simulink model "HIL_model_overall"  (R2014a)
settings: Solver=ode5  StartTime=0.0  StopTime=simulationTime  FixedStep=0.1  RelTol=1e-3
values from neighbouring files (symbols this model uses):
  A_ref = [0.176     0           0 ... (first row only)    [theProgram.m]
  B_ref = [0.0554     0           0 ... (first row only)    [theProgram.m]
  C_ref = [0.05*0.0038     0           0 ... (first row only)    [theProgram.m]
  Di = [50 0 ... (first row only)    [theProgram.m]
  Dist_spv_rfp = sqrt( ( shipL_d(1) - Rfp(1) )^2 + (shipL_d(2) - Rfp(2) )^2 )    [theProgram.m]
  Ds = [-X_u 0 0 ... (first row only)    [theProgram.m]
  iceDiameter = 0.2    [theProgram.m]
  K2_obs = diag([0.25 1 0.5])    [theProgram.m]
  K3_obs = diag([1 1 1])    [theProgram.m]
  K4_obs = diag([250 300 100])    [theProgram.m]
  K_M = [ 1 0 0 ... (first row only)    [theProgram.m]
  K_tow = 20    [theProgram.m]
  kappa = 2    [theProgram.m]
  Kd = [50 0 0 ... (first row only)    [theProgram.m]
  Kp = [10 0 0 ... (first row only)    [theProgram.m]
  Mi_a = iceMass*[1 0; 0 1]    [theProgram.m]
  Mi_rb = iceMass*[1 0; 0 1]    [theProgram.m]
  Ms_a = -[X_udot 0 0 ... (first row only)    [theProgram.m]
  Ms_rb = [shipMass 0 0 ... (first row only)    [theProgram.m]
  Ms_tot = Ms_rb + Ms_a    [theProgram.m]
  Ninstances = 50    [theProgram.m]
  nPoints = size(WP,1)    [theProgram.m]
  Offset_direction = 0    [theProgram.m]
  overturnLimit = 4    [theProgram.m]
  Piceberg = [-4.5; -2.9]    [theProgram.m]
  Pship = [-3.5; -2.9; 0]    [theProgram.m]
  ruptureLimit = 3    [theProgram.m]
  ruptureLimitRef = 9    [theProgram.m]
  ruptureNear = 9.5    [theProgram.m]
  S_trans = [0 -1 0 ... (first row only)    [theProgram.m]
  saved_init = zeros(Ninstances,1)    [theProgram.m]
  sd_break = 0.075*T_break    (= 12)    [theProgram.m]
  sd_overturn = 0.075*T_overturn    (= 9.75)    [theProgram.m]
  sd_slip = 0.075*T_slip    (= 10.5)    [theProgram.m]
  shipL_d = [shipLength-0.55; 0]    [theProgram.m]
  sigma = 0.005    [theProgram.m]
  slippageLimit = 5    [theProgram.m]
  T_bias = diag([20 200 20])    [theProgram.m]
  T_break = 160    [theProgram.m]
  T_overturn = 130    [theProgram.m]
  T_slip = 140    [theProgram.m]
  TowLineLength = 1.11    [theProgram.m]
  u_ref = 0.03    [theProgram.m]
  u_surge_max = 2    [theProgram.m]
  u_sway_max = 1    [theProgram.m]
  u_yaw_max = 2*pi/60    (= 0.10471975512)    [theProgram.m]
  Vc = [cVelocity*cos(cAngle) ... (first row only)    [theProgram.m]
  WP = [-5 -3 ... (first row only)    [theProgram.m]
  WPi_init = 2    [theProgram.m]
libraries: dspmtrx3 x2
(part 2 of 2)

== matlab function HIL_model_overall/LOS controller/LOS iceberg/MATLAB Function1 ==
  data: WPi input; alphaIce input; WP input; WPi_out output; deltaXlos output; eta input; deltaYlos output; WPnormal output; delta output; y_mark output; icebergData input; saved_alphaIce input; alphaIce_save output
function [WPi_out, deltaXlos, deltaYlos, WPnormal, delta, y_mark, alphaIce_save] = fcn(WPi, alphaIce, WP, eta, icebergData, saved_alphaIce)

Lpp = icebergData(1);
n=4;
Rk = 2 * Lpp;

WPi = round(WPi(1));
maxWP = size(WP,1);

x = eta(1);
y = eta(2);

% Delta values
if WPi <= maxWP
    deltaX = WP(WPi,1) - WP(WPi - 1,1);
    deltaY = WP(WPi,2) - WP(WPi - 1,2);
    
    % Switching
    distX = WP(WPi,1) - x;      % Distance to waypoint x-dir
    distY = WP(WPi,2) - y;      % Distance to waypoint y-dir
    if distX^2 + distY^2 <= Rk^2

        WPi = WPi + 1
        if WPi > maxWP
            saved_alphaIce = alphaIce
        end

    end
else
    deltaX = 0;
    deltaY = 0;
    distX = 0;
    distY = 0;
end


% Check if WPi > maxWP
if WPi <= maxWP

    % Calculate LOS
    if abs(deltaX) > 0

        fd = deltaY/deltaX;
        fe = WP(WPi - 1,1);
        ff = WP(WPi - 1,2);
        fg = ff-fd*fe;

        a = 1 + fd^2;
        b = 2*(fd*fg - fd*y - x);
        c = x^2 + y^2 + fg^2 - (n*Lpp)^2 - 2*fg*y;      % Remember n AND Lpp

        fact = -1;
        if deltaX > 0
            fact = 1;
        end

        while (b^2 < 4*a*c)
             n = n+1;
    %         WPi
            c = x^2 + y^2 + fg^2 - (n*Lpp)^2 - 2*fg*y;
        end

        Xlos = (-b + fact*sqrt(b^2 - 4*a*c))/(2*a);
        Ylos = fd*(Xlos - fe) + ff;

    else

        fact = -1;
        if deltaY > 0
            fact = 1;
        end

        Xlos = WP(WPi - 1,1);
        Ylos = y + fact*n*Lpp;

    end

    % Non-current deltaY and deltaX - los
    deltaXlos = Xlos - x;
    deltaYlos = Ylos - y;


    LosPos = sqrt( (Xlos - x)^2 + (Ylos - y)^2 );
    PosOld = sqrt( (x - WP(WPi-1,1))^2 + (y - WP(WPi-1,2))^2 );
    LosOld = sqrt( (Xlos - WP(WPi-1,1))^2 + (Ylos - WP(WPi-1,2))^2 );

    if LosOld == 0
        x_mark = 0;
    else
        x_mark = ( PosOld^2 + LosOld^2 - LosPos^2 ) / ( 2 * LosOld );
    end
    y_mark = sign(PosOld^2 - x_mark^2)*sqrt( abs(PosOld^2 - x_mark^2) );


    % Check if y_mark should be positive of negative by transforming the
    % coordinate system and checking if y-star is positive or negative
    WP_angle = atan2(deltaY,deltaX);
    y_star = -x*sin(WP_angle) + y*cos(WP_angle) + WP(WPi-1,1)*sin(WP_angle) - WP(WPi-1,2)*cos(WP_angle);

    y_mark = -sign(y_star)*y_mark;



    delta = LosOld - x_mark;

    WPnormal = atan2( WP(WPi,2)-WP(WPi-1,2) , WP(WPi,1)-WP(WPi-1,1) ) + pi/2;

    %WPnormal*180/pi

    WPi_out = WPi;

else
    
    WPi_out = WPi;
    deltaXlos = 0;
    deltaYlos = 0;
    WPnormal = 0;
    delta = 0;
    y_mark = 0;
    
end

alphaIce_save = saved_alphaIce;

== matlab function HIL_model_overall/LOS controller/Point Controller,  backstepping/alpha1_dot/MATLAB Function ==
  data: Kp input; z2 input; alpha_1_dot output; z1 input; nu_s input; S input; eta_s input; eta_d input; nu_d input; nu_dot_d input
function alpha_1_dot = fcn(Kp, z2, z1, nu_s, S, eta_s, eta_d, nu_d, nu_dot_d)
%#codegen


if length(eta_s) > 1
    psi_s = eta_s(3);
else
    psi_s = 0;
end
if length(eta_d) > 1
    psi_d = eta_d(3);
else
    psi_d = 0;
end
if length(nu_s) > 1
    rs = nu_s(3);
else
    rs = 0;
end
if length(nu_d) > 1
    rd = nu_d(3);
else
    rd = 0;
end

cs = cos(psi_s);
ss = sin(psi_s);
cd = cos(psi_d);
sd = sin(psi_d);

Rs = [cs -ss 0;
      ss cs 0;
      0 0 1];
Rst = transpose(Rs);
Rd = [cd -sd 0;
      sd cd 0;
      0 0 1];

  
eta_dot_d = Rd*nu_d;
eta_dotdot_d = rd.*Rd*S*nu_d + Rd*nu_dot_d;
alpha_1_dot = -Kp * (z2 - Kp*z1 - rs.*S*z1) - rs.*S*Rst*eta_dot_d + Rst*eta_dotdot_d;

== matlab function HIL_model_overall/LOS controller/Point Controller,  backstepping/Tau/MATLAB Function ==
  data: z1 input; Kd input; z2 input; tau output; D input; nu_s input; eta_s input; b_s input; M input; alpha1_dot input; a output; b output; c output; d output; e output
function [tau, a, b, c, d, e] = fcn(z1, Kd, z2, D, nu_s, eta_s, b_s, M, alpha1_dot)
%#codegen

if length(eta_s) > 1
    psi_s = eta_s(3);
else
    psi_s = 0;
end
if length(nu_s) == 1
    nu_ship = nu_s;
else
    nu_ship = [0;0;0];
end

cs = cos(psi_s);
ss = sin(psi_s);

Rs = [cs -ss 0;
      ss cs 0;
      0 0 1];
Rst = transpose(Rs);

a = z1;
b = Kd*z2;
c = D*nu_ship;
d = Rst*b_s;
e = M*alpha1_dot;
tau = -a -b +c +d +e;

== matlab function HIL_model_overall/LOS controller/Point Controller,  backstepping/alpha_1/MATLAB Function ==
  data: Kp input; alpha_1 output; z1 input; nu_d input; eta_s input; eta_d input
function alpha_1 = fcn(Kp, z1, nu_d, eta_s, eta_d)
%#codegen


if length(eta_d) > 1
    psi_d = eta_d(3);
else
    psi_d = 0;
end
if length(eta_s) > 1
    psi_s = eta_s(3);
else
    psi_s = 0;
end

cd = cos(psi_d);
sd = sin(psi_d);
Rd = [cd -sd 0;
      sd cd 0;
      0 0 1];
  
cs = cos(psi_s);
ss = sin(psi_s);
Rs = [cs -ss 0;
      ss cs 0;
      0 0 1];
Rst = transpose(Rs);

alpha_1 = -Kp * z1 + Rst*Rd*nu_d;

== matlab function HIL_model_overall/LOS controller/Point Controller,  backstepping/z1/R(psi)1 ==
  data: eta input; R output
function R = fcn(eta)

if length(eta) > 1
    psi = eta(3);
else
    psi = 0;
end

c = cos(psi);
s = sin(psi);

R = [c -s 0;
     s c 0;
     0 0 1];

== matlab function HIL_model_overall/LOS controller/Point Controller,  backstepping/z2/MATLAB Function ==
  data: nu_ship input; z2 output; alpha1 input
function z2 = fcn(nu_ship, alpha1)
%#codegen


if length(nu_ship) > 1
    nu_s = nu_ship;
else
    nu_s = [0;0;0];
end

z2 = nu_s - alpha1;

== matlab function HIL_model_overall/LOS controller/Reference Model/Position and attitude reference model/Saturation velocity ==
  data: in input; velMax input; y output; eta_ship input
function y = fcn(in, velMax, eta_ship)
%#codegen

% Check size of u
theSize = length(in);
if theSize < 3
    u = zeros(3,1);
else
    u = in;
end

psi = eta_ship(3);
uMax = velMax(1);
vMax = velMax(2);
psiMax = velMax(3);

xVel = u(1);
yVel = u(2);
r = u(3);

surge = xVel * cos(psi) + yVel * sin(psi);
sway = - xVel * sin(psi) + yVel * cos(psi);
yaw = r;

if abs(surge) > uMax
    surge = sign(surge)*uMax;
end
if abs(sway) > vMax
    sway = sign(sway)*vMax;
end
if abs(yaw) > psiMax
    yaw = sign(yaw)*psiMax;
end

y = u;
y(1) = cos(psi)*surge - sin(psi)*sway;
y(2) = sin(psi)*surge + cos(psi)*sway;
y(3) = yaw;

== matlab function HIL_model_overall/LOS controller/Reference Model/Position and attitude reference model/transformation matrix ==
  data: eta_d_dot input; nu_d output; eta_d_dotdot input; eta_ship input; nu_ship input; nu_dot_d output
function [nu_d,nu_dot_d] = fcn(eta_d_dot, eta_d_dotdot, eta_ship, nu_ship)
%#codegen

psi = eta_ship(3);
r = nu_ship(3);

c = cos(psi);
s = sin(psi);
R_rev = [c s 0;
         -s c 0;
         0 0 1];

nu_d = R_rev * eta_d_dot;

R_rev2 = [0 r 0; -r 0 0; 0 0 0];

nu_dot_d = R_rev * eta_d_dotdot + R_rev2 * nu_d;

== matlab function HIL_model_overall/Nonlinear Passive Observer Towing vessel/estimation/MATLAB Function ==
  data: eta_s_in input; Rs output; Rst output
function [Rs, Rst] = fcn(eta_s_in)

if length(eta_s_in) > 1
    eta_s = eta_s_in;
else
    eta_s = [0; 0; 0];
end

psi = eta_s(3);

c = cos(psi);
s = sin(psi);

Rs = [c -s 0;
      s c 0;
      0 0 1];
Rst = transpose(Rs);

== matlab function HIL_model_overall/Nonlinear Passive Observer Towing vessel/estimation/dead reckoning? ==
  data: eta_s input; eta_s_use output; eta_s_obs input; QS_error input; eta_s_err output
function [eta_s_use, eta_s_err] = fcn(eta_s, eta_s_obs, QS_error)


if QS_error == 0
    eta_s_err = eta_s - eta_s_obs;
    eta_s_use = eta_s;
else
    eta_s_err = [0; 0; 0];
    eta_s_use = eta_s_obs;
end

== matlab function HIL_model_overall/LOS controller/Reference Model/Reference models/Initiation system, try to DP at point some deg out from the WP-start/MATLAB Function ==
  data: WP input; eta_ref output; L_rope input; L_fast input; Offset_direction input
function eta_ref = fcn(WP, L_rope, L_fast, Offset_direction)
%#codegen

x1 = WP(1,1);
y1 = WP(1,2);

x2 = WP(2,1);
y2 = WP(2,2);

beta = atan2(y2-y1,x2-x1);
alpha = beta + Offset_direction * pi/10;    % some degree difference

L = L_rope + L_fast;
x = L*cos(alpha) + x1;
y = L*sin(alpha) + y1;
psi = alpha;

eta_ref = [x; y; psi];

== matlab function HIL_model_overall/LOS controller/Reference Model/Reference models/desired unreferenced ship position/pi -> inf ==
  data: alpha_pi input; alpha_inf output; accumulation input
function alpha_inf  = fcn(alpha_pi, accumulation)


alpha_inf = alpha_pi;
while abs(accumulation - alpha_inf) > pi
    
    sgn = sign(accumulation - alpha_inf);
    alpha_inf = alpha_inf + sgn*2*pi;
    
end

== matlab function HIL_model_overall/LOS controller/Reference Model/Reference models/Velocity reference/delta_T penalty/MATLAB Function ==
  data: deltaT input; out output; delta_lim input; delta_care input
function out = fcn(deltaT, delta_lim, delta_care)
%#eml

if delta_lim ~= delta_care
    a_delta = 1/(delta_lim - delta_care);
    b_delta = -a_delta*delta_care;

    out = a_delta*deltaT + b_delta;
else
    out = 0;
end

== matlab function HIL_model_overall/LOS controller/Reference Model/Reference models/Velocity reference/MATLAB Function1 ==
  data: U_in input; U_ref output; t input
function U_ref = fcn(U_in, t)
%#codegen

% Kick in fully after 100 seconds
U_ref = min(U_in, U_in*t/200);

== matlab function HIL_model_overall/LOS controller/Reference Model/Reference models/Velocity reference/delta_T penalty/Change limiter ==
  data: pen input; newPen output; prevPen input
function newPen = fcn(pen, prevPen)
%#codegen

% pen and prevPen are between 0 and 100

% At prevPen=0, newPen is only allowed to rise by lowLim %/s
lowLim = 1/600000;      % percent rise per second
% At prevPen=100, newPen is only allowed to rise by highLim %/s
highLim = 1/6000;

% newPen is always allowed to decrease, for safety
if pen < prevPen
    newPen = pen;
else
    
    
    % setup for f(x) = ax+b for the rise of newPen
    %   first, convert to %/(s/10)
    lowLim = lowLim/10;
    highLim = highLim/10;
    %   Then find a and b
    b = lowLim;
    a = (highLim - b)/1;
    % Then calculate f(x), which is the maximum rise of the penalty
    % percentage
    maxRise = a*prevPen + b;
    
    newPen = min(prevPen+maxRise, pen);
    
    
end

== matlab function HIL_model_overall/LOS controller/Reference Model/Reference models/End system, after last WP is reached /MATLAB Function ==
  data: L input; WP input; alphaLOS_saved input; eta_ref_end output; nu_ref_end output
function [eta_ref_end, nu_ref_end] = fcn(L, WP, alphaLOS_saved)


% Calculate position of vessel
nWP = size(WP,1);
xWP = WP(nWP,1);
yWP = WP(nWP,2);

x_ref = xWP + L*cos(alphaLOS_saved);
y_ref = yWP + L*sin(alphaLOS_saved);
psi_ref = alphaLOS_saved;

eta_ref_end = [x_ref;
               y_ref;
               psi_ref];
nu_ref_end = [0; 0; 0];

== matlab function HIL_model_overall/LOS controller/Reference Model/Position and attitude reference model/MATLAB Function ==
  data: eta_ref input; eta_dot_ref output; nu_ref input
function eta_dot_ref = fcn(eta_ref, nu_ref)

if length(eta_ref) > 1
    psi_ref = eta_ref(3);
else
    psi_ref = 0;
end

if length(nu_ref) > 1
    nuRef = nu_ref;
else
    nuRef = [0; 0; 0];
end

c = cos(psi_ref);
s = sin(psi_ref);
R = [c -s 0;
     s c 0;
     0 0 1];

eta_dot_ref = R*nuRef;

== matlab function HIL_model_overall/LOS controller/Reference Model/Reference models/Velocity reference/MATLAB Function ==
  data: U input; surge output; eta_ship input; alpha_LOS input; sway output
function [surge, sway] = fcn(U, eta_ship, alpha_LOS)

psi = eta_ship(3);
gamma = alpha_LOS - psi;

surge = U*cos(gamma);
sway = U*sin(gamma);

== matlab function HIL_model_overall/LOS controller/Reference Model/Reference switching/MATLAB Function ==
  data: eta_ini input; eta_out output; nu_ini input; eta input; nu input; eta_end input; nu_end input; time input; nu_out output; WPi input; nWP input
function [eta_out, nu_out] = fcn(eta_ini, nu_ini, eta, nu, eta_end, nu_end, time, WPi, nWP)
%#codegen

switchTime = 10;        % Switch after this many seconds
switchDur = 5;         % Spend this much time switching


if WPi <= nWP

    if time < switchTime

        eta_out = eta_ini;
        nu_out = nu_ini;

    elseif time > switchTime + switchDur || switchTime + switchDur == 0

        eta_out = eta;
        nu_out = nu;

    else

        ini_gain = 1 - (1/switchDur)*( time - switchTime );
        reg_gain = (1/switchDur)*( time - switchTime );

        eta_out = ini_gain * eta_ini + reg_gain * eta;
        nu_out = ini_gain * nu_ini + reg_gain * nu;

    end
    
else
    
    eta_out = eta_end;
    nu_out = nu_end;
    
end
